simulink model "verification_surf"  (R2015b)
settings: Solver=VariableStepAuto  StartTime=0.0  StopTime=inf  RelTol=1e-3
values from neighbouring files (symbols this model uses):
  C = img(max(r2+(c1-1)*sx,1))    [IntegralImage_BoxIntegral_mine.m]
undefined symbols (not defined in the file or in its folder): gray, IsPositionTracked, IsSkeletonTracked, JointDepthIndices, JointImageIndices, JointTrackingState, JointWorldCoordinates, PositionDepthIndices, PositionImageIndices, PositionWorldCoordinates, SegmentationData, SkeletonTrackingID, videoinput
libraries: neural x20, visionsinks x3, visionstatistics x1, imaqlib x1
(part 2 of 5)

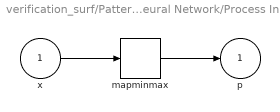
== system verification_surf/Pattern Recognition Neural Network/Process Input 1 ==
  x : Inport  PortDimensions=6912
      mask Display: e = 0.06;c1 = [120 230 180]/255;c2 = ([120 230 180]+0)/(256+128);c3 = ([120 230 180]+128)/(256+128);patch([0 1 1 0],[0 0 1 1],c1);patch([0 1 1 1-e 1-e 0+e],[0 0 1 1-e 0+e 0+e],c2);patch([0 0 1 1-e 0+e 0+e],[0 1 1 1-e 1-e 0+e],c3);plot([0 1 1 0 0],[0 0 1 1 0]);
  mapminmax : neural/Processing Functions/mapminmax  xmin=[-0.033108194499742429;-0.37890545855437574;-0.39483559666479934;-0.4081690237671553;-0.36409218664315945;-0.22851911672555644;-0.13122625820981776;-0.29719658010373889;-0.47795758509560549;-0.42031166340144271;-0.32206314794858759;-0.34976641778690759;-0.11443432644151642;-0.32729044556923326;-0.37684449820299309;-0.34855338542733311;-0.3452064481252155;-0.27454325382897415;-0.12619699116537375;-0.38642723005599122;-0.32171481060704837;-0.41428342330120738;-0.41480878582374564;-0.3010546453027475;-0.087236251452929889;-0.32421386913929062;-0.31728027016626958;-0.3672558334420068;-0.44062033451334692;-0.19216702670796207;-0.083245883839187393;-0.19559032409756658;-0.22006973979435629;-0.39670352712874968;-0.22751316440183464;-0.16245570364994202;-0.1345076062430349;-0.11267643147552679;-0.20000308714623014;-0.18038393453884183;-0.2147763933744993;-0.14780031796605503;-0.28783793746181818;-0.27026120301986062;-0.40275615047118901;-0.43067215275732995;-0.34571525719818952;-0.4173582633014381;-0.33751050420384465;-0.30914698511184041;-0.2939263445321938;-0.32510166969662729;-0.28730467554751166;-0.27231703646663052;-0.29530186651498991;-0.41106419350112805;-0.24670130926110315;-0.36301960357776003;-0.2724285966528423;-0.14560243577857579;-0.12589337030085679;-0.19889778017870122;-0.31379754589057862;-0.34769386915060724;-0.28792514338021619;-0.18214332152580437;-0.11279902781114094;-0.16236849294381231;-0.27265028639014138;-0.30348336411626292;-0.28888300283579676;-0.13899674942668616;0.014108115812031993;0.0027660728982898891;0.0042322440452676191;0.0034991064929408913;0.0044538043110744861;0.0017796548658816967;0.045837295657780865;0.0020071557320756757;0.0039402068244565307;0.0045172437682657347;0.0030806756806606292;0.0011157456689274861;0.015304640820437627;0.0024591118867514964;0.0021976973113759096;0.0068347744471022867;0.0028875631391278678;0.0027786910454560172;0.016708387114366053;0.00034510325049430112;0.0051724478996555421;0.0051383495306359999;0.001146599421663067;0.0023974226702852177;0.019962453910146262;0.00035724308236509243;0.0026401313655217635;0.0024373163727848387;0.0033767977984578662;0.0033969410606259159;0.028753705325125205;0.00043435984232024469;0.0036822288683392018;0.0025440581520558216;0.0013757869750728327;0.0026757989853866565;0.014067555887849241;0.055147234930492284;0.023925386291122622;0.011867841976084511;0.01517776411392595;0.012868202456915404;0.00043047894875815405;0.0026546951232380577;0.0024665334088422274;0.0038693321289044874;0.0029826095948381351;0.0019872432733499851;2.3434656479940881e-14;0.00047289230400833981;0.0046531322471127651;0.0067965966469160817;0.0021709445887244765;8.1651083151617314e-06;4.7058410971405746e-15;0.00094827816765839258;0.0043931402718897566;0.0047142546542418336;0.00017759285022632128;0.0011268328974302769;0;0.0013522512263389548;0.0034505287257270371;0.0064188280190583692;0.0015279164267801057;0.0016048979020984559;7.2357690461092925e-16;0.00034607200448991593;0.0030671665690004467;0.0024019299694261398;0.0021064618954674684;0.00017969163623851819;-0.18722920326823081;-0.27760244395213041;-0.30579128087993757;-0.27200154046185077;-0.27813245637752698;-0.25916729309658487;-0.25336127170767742;-0.34902147496542479;-0.32225272389077092;-0.35489034330226066;-0.28090244072786574;-0.27457520037073802;-0.30683992141310917;-0.30501197735396884;-0.38866261089284493;-0.31254898852828383;-0.31205070526593687;-0.2397475727629135;-0.30060595120950767;-0.32159951593423131;-0.2825226971856043;-0.34179918804691234;-0.27904477383406362;-0.25504159305892504;-0.25574049297505275;-0.28282261551313392;-0.30929911061422372;-0.36907556170333328;-0.37092757494751799;-0.27593236864693449;-0.20893199214415484;-0.2411084344627305;-0.2434085491782805;-0.30886978647177354;-0.21583146081069865;-0.27585745153291619;-0.11888522830973364;-0.12869192944409147;-0.21673711088813194;-0.22967914572602072;-0.2307043158195887;-0.16500524335027822;-0.44922748062116918;-0.43492358572594098 ...(+138451 chars)]  xmax=[0.29066618371602265;0.26868433402449943;0.14205597948505699;0.17919552624058371;0.19048613470096509;0.14672299265495059;0.30785619887380622;0.24589135713116483;0.31267355599281232;0.21322896006161582;0.21298653438106196;0.1812495183480744;0.28155840788364206;0.29138751719470024;0.3433281128434777;0.21845509716011691;0.36706407840126704;0.17975553862132992;0.27489123376876734;0.32339422486254882;0.38717999877148956;0.2886379708035885;0.35717644008652633;0.17434073368737729;0.32467433242369842;0.37046196655838864;0.140183369348929;0.28205773534847156;0.42115179730852642;0.18144165633297135;0.17762763875038923;0.13271881869427854;0.13441019147248143;0.1569305908247782;0.16176291070856369;0.14158713275170443;0.22568485917356026;0.31531258821598929;0.27207001794491009;0.31684999856538992;0.28448041381133049;0.12797128457362045;0.21768320640141609;0.19722087265419994;0.26544444745633877;0.22120509492510346;0.25408602137847519;0.15047416670910657;0.12324859847605311;0.3431716129071401;0.35388379623455601;0.20709873125626743;0.18366310848757139;0.12375871318543456;0.2041244671230879;0.41888172274808605;0.34080755608422447;0.23084055878587764;0.26548591701277624;0.091640180780740169;0.22893357900621178;0.36118666169116109;0.24532095095796855;0.31524528430300897;0.40172725496321915;0.182358168788602;0.13883675391216285;0.14709764473626799;0.15714398160477772;0.17408842461140259;0.18035603639484354;0.10612420783570711;0.38198399186598087;0.38077572223733858;0.41775427898436102;0.40837143180430679;0.38805872023373111;0.2947773833475642;0.40446951488398442;0.42290271967946091;0.48516950085910798;0.42339193792344765;0.50696268458945171;0.36173706595444599;0.46952438529432117;0.38147973592900092;0.43026425899951359;0.43510711922904977;0.52774550192295167;0.30975012491644638;0.54094572821178355;0.53749670493703272;0.56060942290188354;0.49812179380540672;0.48955497808700715;0.31289970884455875;0.4143987199455067;0.45265338287056939;0.35404884754092525;0.45449366164594607;0.47922667846901756;0.26974525724799303;0.25644760556600849;0.29916931191895391;0.31179879692872953;0.41301608101860565;0.34975427671510745;0.22862797910505994;0.43797643245306611;0.3796162735400378;0.55846013986601561;0.58755239222733247;0.54522727163110485;0.40031163843178053;0.36001914519646266;0.42748098774616911;0.42345625239777263;0.44392789941163963;0.37075415539884288;0.44298493032172814;0.37151798497015226;0.38841112787170201;0.41611721267589818;0.50422375635629246;0.48360771699032773;0.32474858571447413;0.36961490003134073;0.48792286161883719;0.41621567911742369;0.58365194569159862;0.4225139176052275;0.21706114969507587;0.26485433396551106;0.48520116216461512;0.39520962477950083;0.55945685575930437;0.45093909540901417;0.35285993412823569;0.15763297330786394;0.17935761369237208;0.27930634231115897;0.35452996962259903;0.34407364402500495;0.19018226395416046;0.20799227367861703;0.19195039052184917;0.22524713493831655;0.23224938837152231;0.2529381829984676;0.21573845357587709;0.22921431591115635;0.30524783409103845;0.24150761250643143;0.28074427043442501;0.27628577831605106;0.23619656791074134;0.23427245284112008;0.3452866814298583;0.31051288921862608;0.23710696177421586;0.30173563726017111;0.22369604914791924;0.28391583366900813;0.34391173512842371;0.27990696432251727;0.31409439327962169;0.31473774803939925;0.24475704677133547;0.26867954697700419;0.33310041005706403;0.29252526034449156;0.27134424057136031;0.36237021472291986;0.23196564154882116;0.20241179626360781;0.1289086325772589;0.20480109791572743;0.21491217171594809;0.24804713852805299;0.19675544140797216;0.34587597272702814;0.40894420511723878;0.42620558636150407;0.399857412732678;0.4104981899723496;0.18067447935396844;0.32501902258293525;0.41393739843861987;0.38560493273530816;0.33507010854613084;0.26242885774543201;0.17599317803891332;0.32701530401817241;0.40207368117773357;0.39635510549927694;0.28325005699907696;0.21890647570423979;0.19687636983094506;0.36299469223947306;0.40406569186833224 ...(+132315 chars)]  ymin=-1  ymax=1
  p : Outport  PortDimensions=6912
      mask Display: e = 0.06;c1 = [120 230 180]/255;c2 = ([120 230 180]+0)/(256+128);c3 = ([120 230 180]+128)/(256+128);patch([0 1 1 0],[0 0 1 1],c1);patch([0 1 1 1-e 1-e 0+e],[0 0 1 1-e 0+e 0+e],c2);patch([0 0 1 1-e 0+e 0+e],[0 1 1 1-e 1-e 0+e],c3);plot([0 1 1 0 0],[0 0 1 1 0]);
  wires:
  x/1 -> mapminmax/1
  mapminmax/1 -> p/1
